simulink model "QPSK_Rayleigh_Channel"  (Simulink 8.4)
settings: Solver=FixedStepDiscrete  StartTime=0.0  StopTime=10  RelTol=1e-3
PreLoadFcn:
  | bitRate = 500000;
  | bitsPerFrame = 200;
  | maxDopplerShift = 200;
  | delayVector = [0:3]*(4e-6);
  | gainVector = [0:3]*(-3);
  | LOSDopplerShift = 100;
  | KFactor = 10;
libraries: commchan3 x2, commrandsrc2 x1, commutil2 x1, commdigbbndam3 x1
Description:
  | Multipath Fading Channel
  | 
  | To learn about this model, click <a href="matlab: showdemo multipathfading_demo;">here</a>.
CloseFcn:
  | clear bitRate
  | clear bitsPerFrame
  | clear maxDopplerShift
  | clear delayVector
  | clear gainVector
  | clear LOSDopplerShift
  | clear KFactor
settings Model: Creator=The MathWorks Inc.  LastModifiedBy=leixia  ExtModeAutoUpdateStatusClock=off  BufferReuse=off
settings DataIOCC: LimitDataPoints=off  SaveOutput=off  SignalLogging=off  SaveTime=off  SignalLoggingName=multipathSigsOut
settings OptimizationCC: BooleanDataType=off  OptimizeBlockIOStorage=off  BufferReuse=off  GlobalBufferReuse=off  ExpressionFolding=off  LocalBlockOutputs=off  InitFltsAndDblsToZero=on  BufferReusableBoundary=off
settings DebuggingCC: SaveWithParameterizedLinksMsg=none  CheckExecutionContextPreStartOutputMsg=on  CheckExecutionContextRuntimeOutputMsg=on  SignalResolutionControl=TryResolveAllWithWarning  SolverPrmCheckMsg=none  InheritedTsInSrcMsg=none  MultiTaskDSMMsg=warning  MultiTaskCondExecSysMsg=none  SigSpecEnsureSampleTimeMsg=none  BusObjectLabelMismatch=none
settings HardwareCC: TargetUnknown=on
settings ModelReferenceCC: UpdateModelReferenceTargets=IfOutOfDate
settings RTWCC: IncludeERTFirstTime=on
settings GRTTargetCC: TargetFcnLib=ansi_tfl_tmw.mat

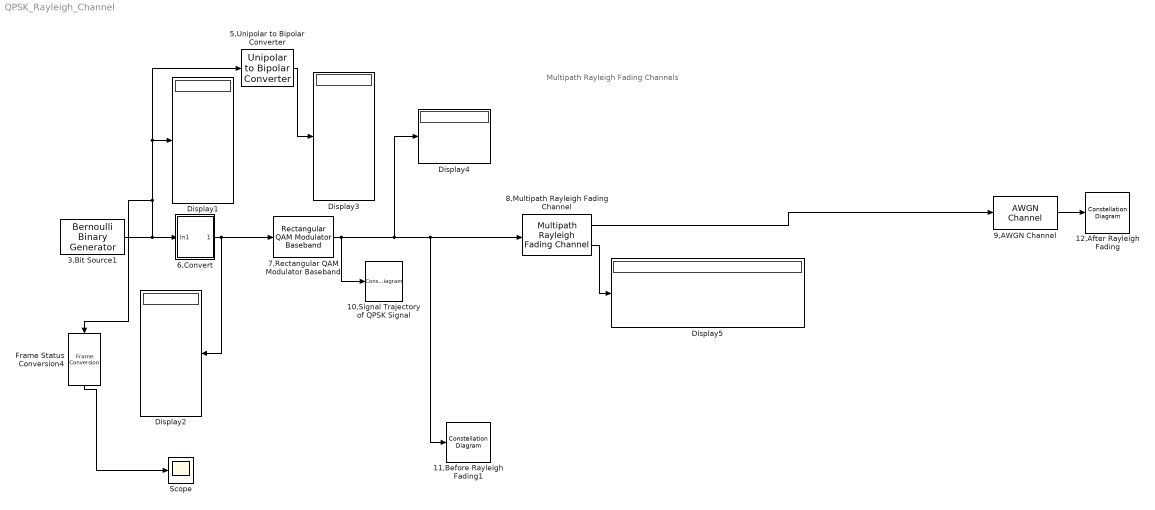
== system QPSK_Rayleigh_Channel ==
  note: Multipath Rayleigh Fading Channels
  10,Signal Trajectory of QPSK Signal : ConstellationDiagram  Tag=SignalTrajectory
  11,Before Rayleigh Fading1 : ConstellationDiagram  Tag=ScatterPlot
  12,After Rayleigh Fading : ConstellationDiagram  Tag=ScatterPlot
  3,Bit Source1 : commrandsrc2/Bernoulli Binary Generator  P=0.5  seed=61  Ts=1/500000  frameBased=on  sampPerFrame=8  orient=off  outDataType=double
  5,Unipolar to Bipolar Converter : commutil2/Unipolar to Bipolar Converter  M=2  polarity=Negative  dataType=Inherit via internal rule
  6,Convert : Subsystem
      mask Display: disp('convert')
  7,Rectangular QAM Modulator Baseband : commdigbbndam3/Rectangular QAM Modulator Baseband  M=4  InType=Bit  Enc=Gray  Mapping=[0,1,2,3]  PowType=Average Power  MinDist=2  AvgPow=1  PeakPow=1  Ph=-pi/2  outDtype=double  outWordLen=16  outUDDataType=sfix(16)  outFracLenMode=Best precision  outFracLen=15
  8,Multipath Rayleigh Fading Channel : commchan3/Multipath Rayleigh Fading Channel  maxDopplerShift=200  spectrumType=Jakes  sigmaGaussian=1/sqrt(2)  coeffRounded=[1 -1.72 0.785]  freqMinMaxRJakes=[0 1]  freqMinMaxAJakes=[0 1]  sigmaGaussian1=1/sqrt(2)  sigmaGaussian2=1/sqrt(2)  centerFreqGaussian1=0.0  centerFreqGaussian2=0.0  gainGaussian1=0.5  gainGaussian2=0.5  coeffBell=9  dopplerSpectrum=doppler.jakes  pathDelays="[ 0    0.0400 ].*1e-4"  avgPathGaindB="[ 0    -3000 ]"  normalizePathGains=on  seed=12345  enableProbe=0  openVisAtStart=on  outPathGains=on  outDelay=off
  9,AWGN Channel : commchan3/AWGN Channel  InputProcessing=Inherited (this choice will be removed - see release notes)  seed=67  noiseMode="Signal to noise ratio  (SNR)"  EbNodB=10  EsNodB=15  SNRdB=200  bitsPerSym=1  Ps=1  Tsym=1e-6  variance=1
  Display{1..5} (5 alike) : Display
  Frame Status Conversion4 : FrameConversion  OutFrame=Sample-based
  Scope : Scope
  wires:
  7,Rectangular QAM Modulator Baseband/1 -> Display4/1, 11,Before Rayleigh Fading1/1, 8,Multipath Rayleigh Fading Channel/1, 10,Signal Trajectory of QPSK Signal/1
  9,AWGN Channel/1 -> 12,After Rayleigh Fading/1
  5,Unipolar to Bipolar Converter/1 -> Display3/1
  6,Convert/1(Out1) -> 7,Rectangular QAM Modulator Baseband/1, Display2/1
  3,Bit Source1/1 -> 6,Convert/1(In1), Display1/1, 5,Unipolar to Bipolar Converter/1, Frame Status Conversion4/1
  8,Multipath Rayleigh Fading Channel/2 -> Display5/1
  8,Multipath Rayleigh Fading Channel/1 -> 9,AWGN Channel/1
  Frame Status Conversion4/1 -> Scope/1

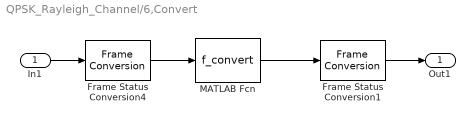
== system QPSK_Rayleigh_Channel/6,Convert ==
  In1 : Inport
  Frame Status Conversion1 : FrameConversion
  Frame Status Conversion4 : FrameConversion  OutFrame=Sample-based
  MATLAB Fcn : MATLABFcn  MATLABFcn=f_convert
  Out1 : Outport
  wires:
  MATLAB Fcn/1 -> Frame Status Conversion1/1
  Frame Status Conversion4/1 -> MATLAB Fcn/1
  In1/1 -> Frame Status Conversion4/1
  Frame Status Conversion1/1 -> Out1/1
